simulink model "deadbeat_running_control"  (R2016b)
settings: configuration reference "Configuration1khz" (kept outside this file)
undefined symbols (not defined in the file or in its folder): A_kalman_no_position, A_kalman_transverse, A_kalman_vertical, A_lpf_accelerometer, A_lpf_contact, A_lpf_imu, A_lpf_lateral_angle, B1_lpf_accelerometer, B1_lpf_contact, B1_lpf_imu, B1_lpf_lateral_angle, B2_lpf_accelerometer, B2_lpf_contact, B2_lpf_imu, B2_lpf_lateral_angle, B_dx_versus_x0, B_kalman_no_position, B_kalman_transverse, B_kalman_vertical, backwards_K_sag_of_t, backwards_P_sag_of_t, C_kalman_no_position, C_kalman_transverse, C_kalman_vertical, com_leg_motor, com_torso, contact_threshold, d_ankle_to_foot, d_vertical_com, desired_com_forward_velocity, desired_com_lateral_velocity, desired_standing_torso_pitch, desired_standing_torso_roll, desired_standing_z, desired_torso_pitch, desired_torso_roll, DiscIntNeverNeededParam, Discrete, enable_bouncing, fdesignblkfcn, flight_duration, forward_dx_of_dxstar, forward_x_of_dxstar, g, gcbh, HIP_MTR_MAX_CONT_TORQUE, HIP_MTR_MAX_TORQUE, i_leg_motor, i_robot, i_torso, initial_dx_estimate, initial_dx_takeoff_history, initial_dx_touchdown_history, initial_dy_estimate, initial_dy_takeoff_history, initial_dy_touchdown_history, initial_dz_estimate, initial_leg_selection, initial_target_dx_history, initial_target_dy_history ... (+80)
libraries: simulink x22, ctrlSharedLib x4, dsparch4 x2
(part 7 of 7)

== matlab function deadbeat_running_control/Behavior/State Estimation/ComputeKneePositions ==
  data: roll input; pitch input; yaw input; left_leg_sagittal_angle input; left_leg_lateral_angle input; left_leg_length input; right_leg_sagittal_angle input; right_leg_lateral_angle input; right_leg_length input; right_back_angle input; left_back_angle input; right_front_angle input; left_front_angle input; m_torso parameter; m_leg_motor parameter; m_leg parameter; com_torso parameter; com_leg_motor parameter; lateral_offset parameter; front_knee_to_right_foot output; back_knee_to_right_foot output; front_knee_to_left_foot output; back_knee_to_left_foot output
function [front_knee_to_right_foot, back_knee_to_right_foot,...
          front_knee_to_left_foot, back_knee_to_left_foot] = ...
         KneePositionsUsingKinematics(roll, pitch, yaw, ...
                                    left_leg_sagittal_angle, left_leg_lateral_angle, left_leg_length, ...
                                    right_leg_sagittal_angle, right_leg_lateral_angle, right_leg_length, ...
                                    right_back_angle, left_back_angle, right_front_angle, left_front_angle,...
                                    m_torso, m_leg_motor, m_leg, com_torso, com_leg_motor, lateral_offset)
                    
    q =  [roll(1), pitch(1), yaw(1), left_leg_sagittal_angle(1), left_leg_lateral_angle(1), left_leg_length(1), right_leg_sagittal_angle(1), right_leg_lateral_angle(1), right_leg_length(1)];
    dq = [roll(2), pitch(2), yaw(2), left_leg_sagittal_angle(2), left_leg_lateral_angle(2), left_leg_length(2), right_leg_sagittal_angle(2), right_leg_lateral_angle(2), right_leg_length(2)];                
    [ ~, ~, left_foot_to_com, ~, right_foot_to_com, ~ ] = ComCalculationFromRobot( q, dq, m_torso, m_leg_motor, m_leg, com_torso, com_leg_motor, lateral_offset );

    q =  [roll(1), pitch(1), yaw(1), left_front_angle(1), left_leg_lateral_angle(1), 0.5, right_front_angle(1), right_leg_lateral_angle(1), 0.5];
    dq = [roll(2), pitch(2), yaw(2), left_front_angle(2), left_leg_lateral_angle(2), 0, right_front_angle(2), right_leg_lateral_angle(2), 0];   
    [ ~, ~, left_front_knee_to_com, ~, right_front_knee_to_com, ~ ] = ComCalculationFromRobot( q, dq, m_torso, m_leg_motor, m_leg, com_torso, com_leg_motor, lateral_offset );
    
    q =  [roll(1), pitch(1), yaw(1), left_back_angle(1), left_leg_lateral_angle(1), 0.4, right_back_angle(1), right_leg_lateral_angle(1), 0.4];
    dq = [roll(2), pitch(2), yaw(2), left_back_angle(2), left_leg_lateral_angle(2), 0, right_back_angle(2), right_leg_lateral_angle(2), 0];   
    [ ~, ~, left_back_knee_to_com, ~, right_back_knee_to_com, ~ ] = ComCalculationFromRobot( q, dq, m_torso, m_leg_motor, m_leg, com_torso, com_leg_motor, lateral_offset );
   
    front_knee_to_left_foot = left_front_knee_to_com(4:6) - left_foot_to_com(4:6);
    front_knee_to_right_foot = right_front_knee_to_com(4:6) - right_foot_to_com(4:6);
    back_knee_to_left_foot = left_back_knee_to_com(4:6) - left_foot_to_com(4:6);
    back_knee_to_right_foot = right_back_knee_to_com(4:6) - right_foot_to_com(4:6);
end

== matlab function deadbeat_running_control/Behavior/State Estimation/Kalman Filtering/Measurement Noise Covariance Matricies ==
  data: R_no_position output; R_transverse output; vertical_GRF_L input; vertical_GRF_R input; R_kalman_foot_stance parameter; R_kalman_foot_slip parameter; R_kalman_accelerometer parameter; R_kalman_dfoot_stance parameter; R_kalman_dfoot_slip parameter; sample_time parameter; m_total_real parameter; g parameter; R_vertical output; kalman_stance_slip_threshold parameter
function [R_no_position, R_transverse, R_vertical] =...
         MeasurementNoiseCovariance(vertical_GRF_L, vertical_GRF_R, ...
           R_kalman_foot_stance, R_kalman_foot_slip, R_kalman_accelerometer, ...
           R_kalman_dfoot_stance, R_kalman_dfoot_slip, ...
           sample_time, m_total_real, g, kalman_stance_slip_threshold)

    % filter states: [dx_w]; [dy_w]; [dz_w];
    % measurements:  [dx_w-dfL + dfL_hat; dx_w-dfR + dfR_hat]; 

    ratio_L = max(0, min(vertical_GRF_L/(kalman_stance_slip_threshold*m_total_real*g),1)); % ratio is 0 if no load, 1 if at least equilibrium
    ratio_R = max(0, min(vertical_GRF_R/(kalman_stance_slip_threshold*m_total_real*g),1));
    R_transverse = diag([ratio_L*R_kalman_foot_stance + (1-ratio_L)*R_kalman_foot_slip, ...
                         ratio_R*R_kalman_foot_stance + (1-ratio_R)*R_kalman_foot_slip, ...
                         R_kalman_accelerometer])/sample_time;
    R_vertical = diag([ratio_L*R_kalman_foot_stance  + (1-ratio_L)*R_kalman_foot_slip,...
                       ratio_R*R_kalman_foot_stance  + (1-ratio_R)*R_kalman_foot_slip,...
                       R_kalman_accelerometer])/sample_time;
                   
    R_no_position = diag([ratio_L*R_kalman_dfoot_stance + (1-ratio_L)*R_kalman_dfoot_slip, ...
                         ratio_R*R_kalman_dfoot_stance + (1-ratio_R)*R_kalman_dfoot_slip, ...
                         R_kalman_accelerometer])/sample_time;
end

== matlab function deadbeat_running_control/Behavior/State Estimation/Kalman Filtering/eigen values ==
  data: Z input; E output
function E = eigen(Z)
    E = real(eig(Z));
    E = sort(E);
end

== matlab function deadbeat_running_control/Behavior/State Estimation/Kalman Filtering/eigen values1 ==
  data: Z input; E output
function E = eigen(Z)
    E = real(eig(Z));
    E = sort(E);
end

== matlab function deadbeat_running_control/Behavior/State Estimation/Kalman Filtering/eigen values2 ==
  data: Z input; E output
function E = eigen(Z)
    E = real(eig(Z));
    E = sort(E);
end

== matlab function deadbeat_running_control/Behavior/State Estimation/PositionUsingRobotGeometry ==
  data: com_left_foot output; dcom_left_foot output; com_right_foot output; dcom_right_foot output; right_left input; horizontal_com_position output; roll input; pitch input; yaw input; horizontal_com_velocity output; lateral_com_position output; lateral_com_velocity output; left_leg_sagittal_angle input; left_leg_lateral_angle input; left_leg_length input; right_leg_sagittal_angle input; right_leg_lateral_angle input; right_leg_length input; m_torso parameter; m_leg_motor parameter; m_leg parameter; com_torso parameter; com_leg_motor parameter; lateral_offset parameter; vertical_com_position output; vertical_com_velocity output; com_pelvis output; dcom_pelvis output
% Returns 2D COM relative to primary foot
function [com_left_foot, dcom_left_foot, com_right_foot, dcom_right_foot,...
          horizontal_com_position, horizontal_com_velocity, ...
          lateral_com_position, lateral_com_velocity, ...
          vertical_com_position, vertical_com_velocity, ...
          com_pelvis, dcom_pelvis] = ...
         ComPositionUsingRobotGeometry(right_left, ...
                                    roll, pitch, yaw, ...
                                    left_leg_sagittal_angle, left_leg_lateral_angle, left_leg_length, ...
                                    right_leg_sagittal_angle, right_leg_lateral_angle, right_leg_length, ...
                                    m_torso, m_leg_motor, m_leg, com_torso, com_leg_motor, lateral_offset)
                    
    q =  [roll(1), pitch(1), yaw(1), left_leg_sagittal_angle(1), left_leg_lateral_angle(1), left_leg_length(1), right_leg_sagittal_angle(1), right_leg_lateral_angle(1), right_leg_length(1)];
    dq = [roll(2), pitch(2), yaw(2), left_leg_sagittal_angle(2), left_leg_lateral_angle(2), left_leg_length(2), right_leg_sagittal_angle(2), right_leg_lateral_angle(2), right_leg_length(2)];
                    
    [ com_pelvis, dcom_pelvis, ...
      com_left_foot, dcom_left_foot, ...
      com_right_foot, dcom_right_foot ] = ...
    ComCalculationFromRobot( q, dq, m_torso, m_leg_motor, m_leg, com_torso, com_leg_motor, lateral_offset );

    if right_left
        com_position = com_right_foot(4:6);
        com_velocity = dcom_right_foot(4:6);
    else
        com_position = com_left_foot(4:6);
        com_velocity = dcom_left_foot(4:6);
    end


    horizontal_com_position = com_position(1);
    horizontal_com_velocity = com_velocity(1);
    lateral_com_position = com_position(2);
    lateral_com_velocity = com_velocity(2);
    vertical_com_position = com_position(3);
    vertical_com_velocity = com_velocity(3);

end
